simulink model "PruebaSensores"  (R2023b)
settings: Solver=VariableStepAuto  StartTime=0.0  StopTime=10.0  RelTol=1e-3
libraries: arduinolib x2
settings Model: Creator=Hajar  LastModifiedBy=Hajar

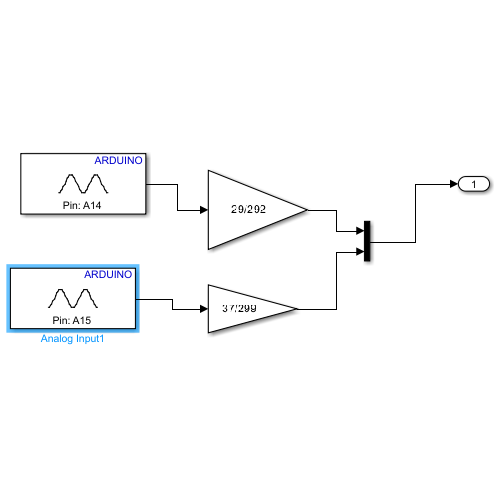
[thumbnail: Simulink's stored preview of the top-level diagram]
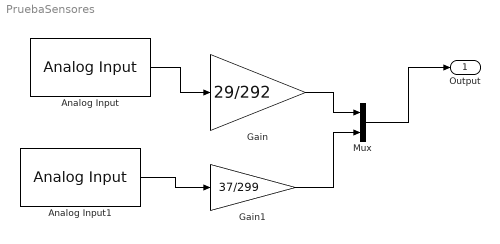
== system PruebaSensores ==
  Analog Input : arduinolib/Analog Input  pinNumber=14  ReadResultsOnly=off  ConversionTriggerSource=Software  ExternalTriggerType=uint32( 0 )  OutputDataType=uint16  EnableConversionCompleteNotify=off  EnableOuputStatus=off  SampleTime=-1  blockPlatform=arduino
  Analog Input1 : arduinolib/Analog Input  pinNumber=15  ReadResultsOnly=off  ConversionTriggerSource=Software  ExternalTriggerType=uint32( 0 )  OutputDataType=uint16  EnableConversionCompleteNotify=off  EnableOuputStatus=off  SampleTime=-1  blockPlatform=arduino
  Gain : Gain  Gain=29/292
  Gain1 : Gain  Gain=37/299
  Mux : Mux  Inputs=2
  Output : Outport
  wires:
  Analog Input1/1 -> Gain1/1
  Analog Input/1 -> Gain/1
  Gain1/1 -> Mux/2
  Gain/1 -> Mux/1
  Mux/1 -> Output/1
